simulink model "TrafficLights"  (R2020b)
settings: Solver=VariableStepAuto  StartTime=0.0  StopTime=10  RelTol=1e-3
settings Model: Creator=sneha  LastModifiedBy=sneha

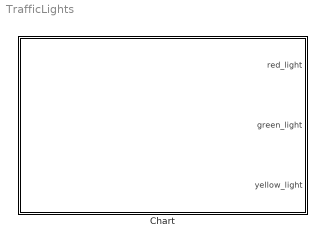
== system TrafficLights ==
  Chart : Stateflow chart  TreatAsAtomicUnit=on

== stateflow chart TrafficLights/Chart ==
  state GoGreen
    entry:
    green_light = 1;
    exit:
    green_light = 0;
  state StopRed
    entry:
    red_light = 1;
    exit:
    red_light = 0;
  state WaitToStop
    state WaitYellow [parallel]
      entry:
      yellow_light = 1;
      exit:
      yellow_light = 0;
      settings: executionOrder=1
    state ToStop [parallel]
      entry:
      green_light = 1;
      exit:
      green_light = 0;
      settings: executionOrder=2
  (default) -> StopRed
  StopRed -> GoGreen : after(5,sec)
  GoGreen -> WaitToStop : after(2,sec)
  WaitToStop -> StopRed : after(1,sec)
  data: red_light output; green_light output; yellow_light output
